simulink model "jam1722"  (R2016a)
settings: Solver=ode23tb  StartTime=0.0  StopTime=2  MaxStep=1e-4  RelTol=1e-3
undefined symbols (not defined in the file): D1, Delta
libraries: powerlib x64, sps_avr x4
settings Model: Creator=eka  LastModifiedBy=willi
settings DataIOCC: SaveFormat=StructureWithTime
settings DebuggingCC: UnconnectedInputMsg=none  UnconnectedOutputMsg=none  UnconnectedLineMsg=none
settings HardwareCC: ProdWordSize=32  ProdHWDeviceType=Specified
settings ConfigComp: CovModelRefEnable=Off

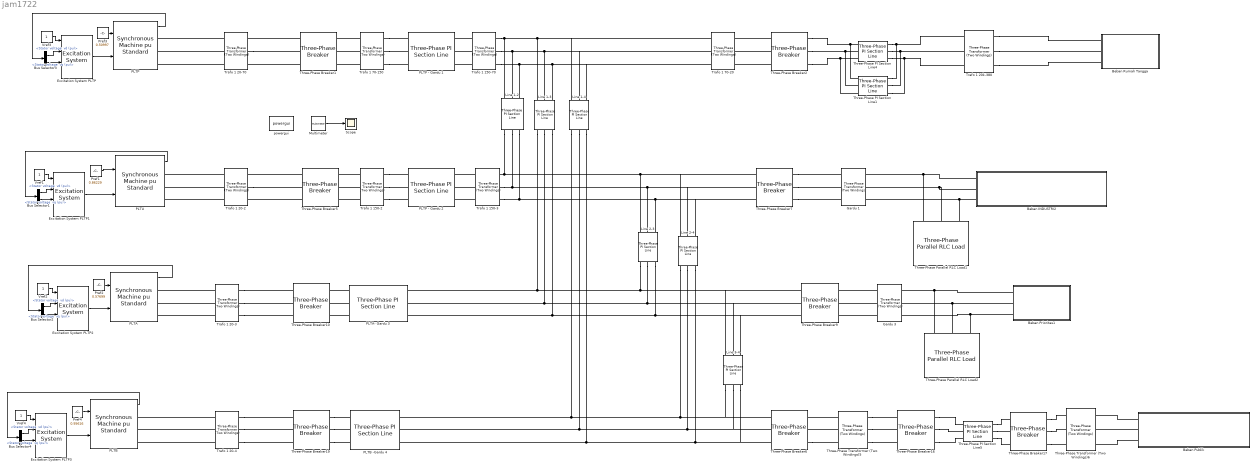
== system jam1722 ==
  Beban INDUSTRI2 : Subsystem
  Beban Prioritas1 : Subsystem
  Beban Publik : Subsystem
  Beban Rumah Tangga : Subsystem
  Bus Selector{1..4} (4 alike) : BusSelector  OutputSignals="dq0 components.Stator voltage  vd (pu),dq0 components.Stator voltage  vq (pu)"
  Excitation System PLTP : sps_avr/Excitation System  tr=20e-3  reg=[ 300, 0.001 ]  exc=[ 1, 0 ]  tgr=[ 0, 0 ]  damp=[ 0.001, 0.1 ]  sat=[ 0, 0 ]  lim=[ -11.5, 11.5, 0 ]  v0=[1 1.2849]
  Excitation System PLTP1 : sps_avr/Excitation System  tr=20e-3  reg=[ 300, 0.001 ]  exc=[ 1, 0 ]  tgr=[ 0, 0 ]  damp=[ 0.001, 0.1 ]  sat=[ 0, 0 ]  lim=[ -11.5, 11.5, 0 ]  v0=[1 1.6958]
  Excitation System PLTP2 : sps_avr/Excitation System  tr=20e-3  reg=[ 300, 0.001 ]  exc=[ 1, 0 ]  tgr=[ 0, 0 ]  damp=[ 0.001, 0.1 ]  sat=[ 0, 0 ]  lim=[ -11.5, 11.5, 0 ]  v0=[1 1.4349]
  Excitation System PLTP3 : sps_avr/Excitation System  tr=20e-3  reg=[ 300, 0.001 ]  exc=[ 1, 0 ]  tgr=[ 0, 0 ]  damp=[ 0.001, 0.1 ]  sat=[ 0, 0 ]  lim=[ -11.5, 11.5, 0 ]  v0=[1 4.931]
  Gardu 1 : powerlib/Elements/Three-Phase Transformer (Two Windings)  Winding1Connection=Yg  Winding2Connection=Delta (D1)  CoreType=Three single-phase transformers  SetSaturation=off  Hysteresis=off  DataFile='hysteresis'  SetInitialFlux=off  Measurements=None  UNITS=pu  NominalPower=[ 250e6 , 50 ]  Winding1=[ 70e3 , 0.005 , 0.0159 ]  Winding2=[ 20e3 , 0.005 , 0]  Rm=500  Lm=500  L0=0.5  Saturation=[ 0,0 ; 0.0024,1.2 ; 1.0,1.52 ]  InitialFluxes=[ 0.8 , -0.8 , 0.7 ]  MoreParameters=off  BreakLoop=off  DataType=off  TransfoNumber=1
  Gardu 3 : powerlib/Elements/Three-Phase Transformer (Two Windings)  Winding1Connection=Yg  Winding2Connection=Delta (D1)  CoreType=Three single-phase transformers  SetSaturation=off  Hysteresis=off  DataFile='hysteresis'  SetInitialFlux=off  Measurements=None  UNITS=pu  NominalPower=[ 250e6 , 50 ]  Winding1=[ 70e3 , 0.005 , 0.0159 ]  Winding2=[20e3 , 0.005 , 0]  Rm=500  Lm=500  L0=0.5  Saturation=[ 0,0 ; 0.0024,1.2 ; 1.0,1.52 ]  InitialFluxes=[ 0.8 , -0.8 , 0.7 ]  MoreParameters=off  BreakLoop=off  DataType=off  TransfoNumber=1
  Line 1-2 : powerlib/Elements/Three-Phase PI Section Line  LConnTagsString=a|b|c  RConnTagsString=A|B|C  Frequency=50  Resistances=[ 0.2 0.3864]  Inductances="[ 0.9337e-3  4.1264e-3]"  Capacitances=[12.74e-9 7.751e-9]  Length=20
  Line 1-3 : powerlib/Elements/Three-Phase PI Section Line  LConnTagsString=a|b|c  RConnTagsString=A|B|C  Frequency=50  Resistances=[ 0.2 0.3864]  Inductances="[ 0.9337e-3  4.1264e-3]"  Capacitances=[12.74e-9 7.751e-9]  Length=5
  Line 1-4 : powerlib/Elements/Three-Phase PI Section Line  LConnTagsString=a|b|c  RConnTagsString=A|B|C  Frequency=50  Resistances=[ 0.2 0.3864]  Inductances="[ 0.9337e-3  4.1264e-3]"  Capacitances=[12.74e-9 7.751e-9]  Length=20
  Line 2-3 : powerlib/Elements/Three-Phase PI Section Line  LConnTagsString=a|b|c  RConnTagsString=A|B|C  Frequency=50  Resistances=[ 0.2 0.3864]  Inductances="[ 0.9337e-3  4.1264e-3]"  Capacitances=[12.74e-9 7.751e-9]  Length=5
  Line 2-4 : powerlib/Elements/Three-Phase PI Section Line  LConnTagsString=a|b|c  RConnTagsString=A|B|C  Frequency=50  Resistances=[ 0.2 0.3864]  Inductances="[ 0.9337e-3  4.1264e-3]"  Capacitances=[12.74e-9 7.751e-9]  Length=20
  Line 3-4 : powerlib/Elements/Three-Phase PI Section Line  LConnTagsString=a|b|c  RConnTagsString=A|B|C  Frequency=50  Resistances=[ 0.2 0.3864]  Inductances="[ 0.9337e-3  4.1264e-3]"  Capacitances=[12.74e-9 7.751e-9]  Length=5
  Multimeter : powerlib/Measurements/Multimeter  PhasorSimulation=off  OutputType=Complex  sel=1  L=1  Gain=0  yselected={}  PSBOutputType=1  PSBequivalent=0  AxesSetting=[0,0.1,-100,100]  Display=0  SavedBlockNames=-11
  PLTA : powerlib/Machines/Synchronous Machine pu Standard  PresetModel=No  MechanicalLoad=Mechanical power Pm  ShowDetailedParameters=on  RotorType=Salient-pole  Units=per unit standard parameters  MeasurementBus=off  NominalParameters=[36e6 20000 50]  Reactances1=[ 1.81, 0.3, 0.23, 1.76, 0.65, 0.25, 0.15 ]  Reactances2=[2.24 0.17 0.12 1.02 0.13 0.08]  dAxisTimeConstants=Short-circuit  qAxisTimeConstants=Short-circuit  TimeConstants1="[ 4.4849  0.0681  0.1  ]"  TimeConstants2=[ 8.0, 0.03, 1.0, 0.07 ]  TimeConstants3="[  4.49  0.0681  0.0513  ]"  TimeConstants4=[ 8.0, 0.03, 0.3371, 0.0295 ]  TimeConstants5=[ 1.01, 0.053, 0.1 ]  TimeConstants6=[ 1.3201, 0.023, 1.0, 0.07 ]  TimeConstants7=[0.012 0.003 0.003]  TimeConstants8=[ 1.3201, 0.0231, 0.3371, 0.0295 ]  StatorResistance=0.037875  Mechanical=[0.1028 0.02056 2]  PolePairs=2  InitialConditions=[0 -59.3108 0.566752 0.566752 0.566752 4.73334 -115.267 124.733 1.43489]  SetSaturation=on  Saturation=[0.6404,0.7127,0.8441,0.9214,0.9956,1.082,1.19,1.316,1.457;0.7,0.7698,0.8872,0.9466,0.9969,1.046,1.1,1.151,1.201]  LoadFlowParameters=[1,0,0,0,0]  TsPowergui=0  TsBlock=-1  IterativeModel=Trapezoidal non iterative  IterativeDiscreteModel=Trapezoidal non iterative  BusType=swing  Pref=0  Qref=0  Qmin=-inf  Qmax=inf  PLF=0  QLF=0
  PLTA- Gardu 3 : powerlib/Elements/Three-Phase PI Section Line  LConnTagsString=a|b|c  RConnTagsString=A|B|C  Frequency=50  Resistances=[ 0.2 0.3864]  Inductances="[ 0.9337e-3  4.1264e-3]"  Capacitances=[12.74e-9 7.751e-9]  Length=50
  PLTB : powerlib/Machines/Synchronous Machine pu Standard  PresetModel=No  MechanicalLoad=Mechanical power Pm  ShowDetailedParameters=on  RotorType=Salient-pole  Units=per unit standard parameters  MeasurementBus=off  NominalParameters=[12e6 20000 50]  Reactances1=[ 1.81, 0.3, 0.23, 1.76, 0.65, 0.25, 0.15 ]  Reactances2=[2.24 0.17 0.12 1.02 0.13 0.08]  dAxisTimeConstants=Short-circuit  qAxisTimeConstants=Short-circuit  TimeConstants1="[ 4.4849  0.0681  0.1  ]"  TimeConstants2=[ 8.0, 0.03, 1.0, 0.07 ]  TimeConstants3="[  4.49  0.0681  0.0513  ]"  TimeConstants4=[ 8.0, 0.03, 0.3371, 0.0295 ]  TimeConstants5=[ 1.01, 0.053, 0.1 ]  TimeConstants6=[ 1.3201, 0.023, 1.0, 0.07 ]  TimeConstants7=[0.012 0.003 0.003]  TimeConstants8=[ 1.3201, 0.0231, 0.3371, 0.0295 ]  StatorResistance=0.037875  Mechanical=[0.1028 0.02056 2]  PolePairs=2  InitialConditions=[0 -77.6086 1.80081 1.80081 1.80081 -66.5761 -186.576 53.4239 4.93097]  SetSaturation=on  Saturation=[0.6404,0.7127,0.8441,0.9214,0.9956,1.082,1.19,1.316,1.457;0.7,0.7698,0.8872,0.9466,0.9969,1.046,1.1,1.151,1.201]  LoadFlowParameters=[1,0,0,0,0]  TsPowergui=0  TsBlock=-1  IterativeModel=Trapezoidal non iterative  IterativeDiscreteModel=Trapezoidal non iterative  BusType=PV  Pref=10e6  Qref=0  Qmin=-inf  Qmax=inf  PLF=0  QLF=0
  PLTB -Gardu 4 : powerlib/Elements/Three-Phase PI Section Line  LConnTagsString=a|b|c  RConnTagsString=A|B|C  Frequency=50  Resistances=[ 0.2 0.3864]  Inductances="[ 0.9337e-3  4.1264e-3]"  Capacitances=[12.74e-9 7.751e-9]  Length=20
  PLTP : powerlib/Machines/Synchronous Machine pu Standard  PresetModel=No  MechanicalLoad=Mechanical power Pm  ShowDetailedParameters=on  RotorType=Salient-pole  Units=per unit standard parameters  MeasurementBus=off  NominalParameters=[96e6 20000 50]  Reactances1=[ 1.81, 0.3, 0.23, 1.76, 0.65, 0.25, 0.15 ]  Reactances2=[2.24 0.17 0.12 1.02 0.13 0.08]  dAxisTimeConstants=Short-circuit  qAxisTimeConstants=Short-circuit  TimeConstants1="[ 4.4849  0.0681  0.1  ]"  TimeConstants2=[ 8.0, 0.03, 1.0, 0.07 ]  TimeConstants3="[  4.49  0.0681  0.0513  ]"  TimeConstants4=[ 8.0, 0.03, 0.3371, 0.0295 ]  TimeConstants5=[ 1.01, 0.053, 0.1 ]  TimeConstants6=[ 1.3201, 0.023, 1.0, 0.07 ]  TimeConstants7=[0.012 0.003 0.003]  TimeConstants8=[ 1.3201, 0.0231, 0.3371, 0.0295 ]  StatorResistance=0.037875  Mechanical=[0.1028 0.02056 2]  PolePairs=2  InitialConditions=[0 -61.4393 0.505842 0.505842 0.505842 8.5019 -111.498 128.502 1.28494]  SetSaturation=on  Saturation=[0.6404,0.7127,0.8441,0.9214,0.9956,1.082,1.19,1.316,1.457;0.7,0.7698,0.8872,0.9466,0.9969,1.046,1.1,1.151,1.201]  LoadFlowParameters=[1,0,0,0,0]  TsPowergui=0  TsBlock=-1  IterativeModel=Trapezoidal non iterative  IterativeDiscreteModel=Trapezoidal non iterative  BusType=swing  Pref=400E6  Qref=0  Qmin=-inf  Qmax=inf  PLF=0  QLF=0
  PLTP - Gardu 1 : powerlib/Elements/Three-Phase PI Section Line  LConnTagsString=a|b|c  RConnTagsString=A|B|C  Frequency=50  Resistances=[ 0.2 0.3864]  Inductances="[ 0.9337e-3  4.1264e-3]"  Capacitances=[12.74e-9 7.751e-9]  Length=100
  PLTP - Gardu 2 : powerlib/Elements/Three-Phase PI Section Line  LConnTagsString=a|b|c  RConnTagsString=A|B|C  Frequency=50  Resistances=[ 0.2 0.3864]  Inductances="[ 0.9337e-3  4.1264e-3]"  Capacitances=[12.74e-9 7.751e-9]  Length=100
  PLTU : powerlib/Machines/Synchronous Machine pu Standard  PresetModel=No  MechanicalLoad=Mechanical power Pm  ShowDetailedParameters=on  RotorType=Salient-pole  Units=per unit standard parameters  MeasurementBus=off  NominalParameters=[120e6 20000 50]  Reactances1=[ 1.81, 0.3, 0.23, 1.76, 0.65, 0.25, 0.15 ]  Reactances2=[2.24 0.17 0.12 1.02 0.13 0.08]  dAxisTimeConstants=Short-circuit  qAxisTimeConstants=Short-circuit  TimeConstants1="[ 4.4849  0.0681  0.1  ]"  TimeConstants2=[ 8.0, 0.03, 1.0, 0.07 ]  TimeConstants3="[  4.49  0.0681  0.0513  ]"  TimeConstants4=[ 8.0, 0.03, 0.3371, 0.0295 ]  TimeConstants5=[ 1.01, 0.053, 0.1 ]  TimeConstants6=[ 1.3201, 0.023, 1.0, 0.07 ]  TimeConstants7=[0.012 0.003 0.003]  TimeConstants8=[ 1.3201, 0.0231, 0.3371, 0.0295 ]  StatorResistance=0.037875  Mechanical=[0.1028 0.02056 2]  PolePairs=2  InitialConditions=[0 -93.9732 0.874366 0.874366 0.874366 -34.8255 -154.826 85.1745 1.69579]  SetSaturation=on  Saturation=[0.6404,0.7127,0.8441,0.9214,0.9956,1.082,1.19,1.316,1.457;0.7,0.7698,0.8872,0.9466,0.9969,1.046,1.1,1.151,1.201]  LoadFlowParameters=[1,0,0,0,0]  TsPowergui=0  TsBlock=-1  IterativeModel=Trapezoidal non iterative  IterativeDiscreteModel=Trapezoidal non iterative  BusType=PV  Pref=100e6  Qref=0  Qmin=-inf  Qmax=inf  PLF=0  QLF=0
  Pref1 : Constant  Value=0.86229
  Pref2 : Constant  Value=0.57699
  Pref3 : Constant  Value=0.50997
  Pref4 : Constant  Value=0.95616
  Scope : Scope
  Three-Phase PI Section Line1 : powerlib/Elements/Three-Phase PI Section Line  LConnTagsString=a|b|c  RConnTagsString=A|B|C  Frequency=50  Resistances=[ 0.2 0.3864]  Inductances="[ 0.9337e-3  4.1264e-3]"  Capacitances=[12.74e-9 7.751e-9]  Length=3
  Three-Phase PI Section Line4 : powerlib/Elements/Three-Phase PI Section Line  LConnTagsString=a|b|c  RConnTagsString=A|B|C  Frequency=50  Resistances=[ 0.2 0.3864]  Inductances="[ 0.9337e-3  4.1264e-3]"  Capacitances=[12.74e-9 7.751e-9]  Length=3
  Three-Phase PI Section Line5 : powerlib/Elements/Three-Phase PI Section Line  LConnTagsString=a|b|c  RConnTagsString=A|B|C  Frequency=50  Resistances=[ 0.2 0.3864]  Inductances="[ 0.9337e-3  4.1264e-3]"  Capacitances=[12.74e-9 7.751e-9]  Length=3
  Three-Phase Parallel RLC Load1 : powerlib/Elements/Three-Phase Parallel RLC Load  LConnTagsString=A|B|C  Configuration=Delta  NominalVoltage=380  Vabc=[1e3 1e3 1e3]  Vabcp=[1e3 1e3 1e3]  NominalFrequency=50  UnbalancedPower=off  ActivePower=0  InductivePower=0  CapacitivePower=35000  Pabc=[10e3 9e3 11e3]  QLabc=[100 90 110]  QCabc=[100 90 110]  Pabcp=[10e3 9e3 11e3]  QLabcp=[100 90 110]  QCabcp=[100 90 110]  Measurements=None  LoadType=constant Z
  Three-Phase Parallel RLC Load2 : powerlib/Elements/Three-Phase Parallel RLC Load  LConnTagsString=A|B|C  Configuration=Delta  NominalVoltage=380  Vabc=[1e3 1e3 1e3]  Vabcp=[1e3 1e3 1e3]  NominalFrequency=50  UnbalancedPower=off  ActivePower=0  InductivePower=0  CapacitivePower=10000  Pabc=[10e3 9e3 11e3]  QLabc=[100 90 110]  QCabc=[100 90 110]  Pabcp=[10e3 9e3 11e3]  QLabcp=[100 90 110]  QCabcp=[100 90 110]  Measurements=None  LoadType=constant Z
  Three-Phase Transformer (Two Windings)5 : powerlib/Elements/Three-Phase Transformer (Two Windings)  Winding1Connection=Delta (D1)  Winding2Connection=Yg  CoreType=Three single-phase transformers  SetSaturation=off  Hysteresis=off  DataFile='hysteresis'  SetInitialFlux=off  Measurements=None  UNITS=pu  NominalPower=[ 250e6 , 50 ]  Winding1=[70e3 , 0.005 , 0 ]  Winding2=[20e3 , 0.005 , 0.0159 ]  Rm=500  Lm=500  L0=0.5  Saturation=[ 0,0 ; 0.0024,1.2 ; 1.0,1.52 ]  InitialFluxes=[ 0.8 , -0.8 , 0.7 ]  MoreParameters=off  BreakLoop=off  DataType=off  TransfoNumber=1
  Three-Phase Transformer (Two Windings)6 : powerlib/Elements/Three-Phase Transformer (Two Windings)  Winding1Connection=Yg  Winding2Connection=Delta (D1)  CoreType=Three single-phase transformers  SetSaturation=off  Hysteresis=off  DataFile='hysteresis'  SetInitialFlux=off  Measurements=None  UNITS=pu  NominalPower=[ 220e6 , 50 ]  Winding1=[ 20e3 , 0.005 , 0.0159 ]  Winding2=[ 380 , 0.005 , 0]  Rm=500  Lm=500  L0=0.5  Saturation=[ 0,0 ; 0.0024,1.2 ; 1.0,1.52 ]  InitialFluxes=[ 0.8 , -0.8 , 0.7 ]  MoreParameters=off  BreakLoop=off  DataType=off  TransfoNumber=1
  Three-Phase Breaker{1,5..7,9..10,16..17,19} (9 alike) : powerlib/Elements/Three-Phase Breaker  InitialState=closed  SwitchA=off  SwitchB=off  SwitchC=off  SwitchTimes="[1/60  5/60]"  External=off  BreakerResistance=0.01  SnubberResistance=1e6  SnubberCapacitance=inf  Measurements=None
  Three-Phase Breaker2 : powerlib/Elements/Three-Phase Breaker  InitialState=closed  SwitchA=off  SwitchB=off  SwitchC=off  SwitchTimes="[1/60  5/60]"  External=off  BreakerResistance=0.0005  SnubberResistance=1e6  SnubberCapacitance=inf  Measurements=None
  Trafo 1 150-2 : powerlib/Elements/Three-Phase Transformer (Two Windings)  Winding1Connection=Yg  Winding2Connection=Delta (D1)  CoreType=Three single-phase transformers  SetSaturation=off  Hysteresis=off  DataFile='hysteresis'  SetInitialFlux=off  Measurements=None  UNITS=pu  NominalPower=[ 250e6 , 50 ]  Winding1=[70e3 , 0.005 , 0]  Winding2="[150e3 , 0.005 , 0.0159  ]"  Rm=500  Lm=500  L0=0.5  Saturation=[ 0,0 ; 0.0024,1.2 ; 1.0,1.52 ]  InitialFluxes=[ 0.8 , -0.8 , 0.7 ]  MoreParameters=off  BreakLoop=off  DataType=off  TransfoNumber=1
  Trafo 1 150-3 : powerlib/Elements/Three-Phase Transformer (Two Windings)  Winding1Connection=Delta (D1)  Winding2Connection=Yg  CoreType=Three single-phase transformers  SetSaturation=off  Hysteresis=off  DataFile='hysteresis'  SetInitialFlux=off  Measurements=None  UNITS=pu  NominalPower=[ 250e6 , 50 ]  Winding1=[150e3 , 0.005 , 0.0159 ]  Winding2=[70e3 , 0.005 , 0 ]  Rm=500  Lm=500  L0=0.5  Saturation=[ 0,0 ; 0.0024,1.2 ; 1.0,1.52 ]  InitialFluxes=[ 0.8 , -0.8 , 0.7 ]  MoreParameters=off  BreakLoop=off  DataType=off  TransfoNumber=1
  Trafo 1 150-70 : powerlib/Elements/Three-Phase Transformer (Two Windings)  Winding1Connection=Yg  Winding2Connection=Delta (D1)  CoreType=Three single-phase transformers  SetSaturation=off  Hysteresis=off  DataFile='hysteresis'  SetInitialFlux=off  Measurements=None  UNITS=pu  NominalPower=[ 250e6 , 50 ]  Winding1=[150e3 , 0.005 , 0.0159 ]  Winding2=[70e3 , 0.005 , 0 ]  Rm=500  Lm=500  L0=0.5  Saturation=[ 0,0 ; 0.0024,1.2 ; 1.0,1.52 ]  InitialFluxes=[ 0.8 , -0.8 , 0.7 ]  MoreParameters=off  BreakLoop=off  DataType=off  TransfoNumber=1
  Trafo 1 20-2 : powerlib/Elements/Three-Phase Transformer (Two Windings)  Winding1Connection=Delta (D1)  Winding2Connection=Yg  CoreType=Three single-phase transformers  SetSaturation=off  Hysteresis=off  DataFile='hysteresis'  SetInitialFlux=off  Measurements=None  UNITS=pu  NominalPower=[ 210e6 , 50 ]  Winding1=[20e3 , 0.005 , 0.0159 ]  Winding2=[70e3 , 0.005 , 0 ]  Rm=500  Lm=500  L0=0.5  Saturation=[ 0,0 ; 0.0024,1.2 ; 1.0,1.52 ]  InitialFluxes=[ 0.8 , -0.8 , 0.7 ]  MoreParameters=off  BreakLoop=off  DataType=off  TransfoNumber=1
  Trafo 1 20-3 : powerlib/Elements/Three-Phase Transformer (Two Windings)  Winding1Connection=Yg  Winding2Connection=Delta (D1)  CoreType=Three single-phase transformers  SetSaturation=off  Hysteresis=off  DataFile='hysteresis'  SetInitialFlux=off  Measurements=None  UNITS=pu  NominalPower=[ 210e6 , 50 ]  Winding1=[20e3 , 0.005 , 0.0159 ]  Winding2=[70e3 , 0.005 , 0 ]  Rm=500  Lm=500  L0=0.5  Saturation=[ 0,0 ; 0.0024,1.2 ; 1.0,1.52 ]  InitialFluxes=[ 0.8 , -0.8 , 0.7 ]  MoreParameters=off  BreakLoop=off  DataType=off  TransfoNumber=1
  Trafo 1 20-4 : powerlib/Elements/Three-Phase Transformer (Two Windings)  Winding1Connection=Yg  Winding2Connection=Delta (D1)  CoreType=Three single-phase transformers  SetSaturation=off  Hysteresis=off  DataFile='hysteresis'  SetInitialFlux=off  Measurements=None  UNITS=pu  NominalPower=[ 210e6 , 50 ]  Winding1=[20e3 , 0.005 , 0.0159 ]  Winding2=[70e3 , 0.005 , 0 ]  Rm=500  Lm=500  L0=0.5  Saturation=[ 0,0 ; 0.0024,1.2 ; 1.0,1.52 ]  InitialFluxes=[ 0.8 , -0.8 , 0.7 ]  MoreParameters=off  BreakLoop=off  DataType=off  TransfoNumber=1
  Trafo 1 20-70 : powerlib/Elements/Three-Phase Transformer (Two Windings)  Winding1Connection=Yg  Winding2Connection=Delta (D1)  CoreType=Three single-phase transformers  SetSaturation=off  Hysteresis=off  DataFile='hysteresis'  SetInitialFlux=off  Measurements=None  UNITS=pu  NominalPower=[ 210e6 , 50 ]  Winding1=[20e3 , 0.005 , 0.0159 ]  Winding2=[70e3 , 0.005 , 0 ]  Rm=500  Lm=500  L0=0.5  Saturation=[ 0,0 ; 0.0024,1.2 ; 1.0,1.52 ]  InitialFluxes=[ 0.8 , -0.8 , 0.7 ]  MoreParameters=off  BreakLoop=off  DataType=off  TransfoNumber=1
  Trafo 1 20k-380 : powerlib/Elements/Three-Phase Transformer (Two Windings)  Winding1Connection=Yg  Winding2Connection=Delta (D1)  CoreType=Three single-phase transformers  SetSaturation=off  Hysteresis=off  DataFile='hysteresis'  SetInitialFlux=off  Measurements=None  UNITS=pu  NominalPower=[ 220e6 , 50 ]  Winding1="[ 18000, 0.005 ,0.0159  ]"  Winding2=[ 380 , 0.005 , 0]  Rm=500  Lm=500  L0=0.5  Saturation=[ 0,0 ; 0.0024,1.2 ; 1.0,1.52 ]  InitialFluxes=[ 0.8 , -0.8 , 0.7 ]  MoreParameters=off  BreakLoop=off  DataType=off  TransfoNumber=1
  Trafo 1 70-150 : powerlib/Elements/Three-Phase Transformer (Two Windings)  Winding1Connection=Delta (D1)  Winding2Connection=Yg  CoreType=Three single-phase transformers  SetSaturation=off  Hysteresis=off  DataFile='hysteresis'  SetInitialFlux=off  Measurements=None  UNITS=pu  NominalPower=[ 250e6 , 50 ]  Winding1=[70e3 , 0.005 , 0]  Winding2="[150e3 , 0.005 , 0.0159  ]"  Rm=500  Lm=500  L0=0.5  Saturation=[ 0,0 ; 0.0024,1.2 ; 1.0,1.52 ]  InitialFluxes=[ 0.8 , -0.8 , 0.7 ]  MoreParameters=off  BreakLoop=off  DataType=off  TransfoNumber=1
  Trafo 1 70-20 : powerlib/Elements/Three-Phase Transformer (Two Windings)  Winding1Connection=Delta (D1)  Winding2Connection=Yg  CoreType=Three single-phase transformers  SetSaturation=off  Hysteresis=off  DataFile='hysteresis'  SetInitialFlux=off  Measurements=None  UNITS=pu  NominalPower=[ 220e6 , 50 ]  Winding1=[70e3 , 0.005 , 0 ]  Winding2=[20e3 , 0.005 , 0.0159 ]  Rm=500  Lm=500  L0=0.5  Saturation=[ 0,0 ; 0.0024,1.2 ; 1.0,1.52 ]  InitialFluxes=[ 0.8 , -0.8 , 0.7 ]  MoreParameters=off  BreakLoop=off  DataType=off  TransfoNumber=1
  Vref{1..4} (4 alike) : Constant
  powergui : powerlib/powergui  Priority=1  SimulationMode=Continuous  SolverType=Tustin  SampleTime=50e-6  frequency=60  SPID=on  DisableSnubberDevices=off  DisableRonSwitches=off  DisableVfSwitches=off  SwTol=0  DisplayEquations=off  Interpol=off  ExternalGateDelay=off  methode=off  Ts=100  FunctionMessages=off  echomessages=off  HookPort=off  EnableUseOfTLC=off  x0status=blocks  frequencyindice=50  Pbase=100e6  ErrMax=0.0001  Iterations=300  UnitsV=kV  UnitsW=MW  buscounter=0  RestoreLinks=warning  ResistiveCurrentMeasurement=off  Frange=[0:2:500]  Ylog=off  Xlog=on  ShowGrid=off  save=off  variable=ZData  structure=0  ZoomFFT=off  StartTime=0.0  cycles=1  DisplayStyle=1  fundamental=60  FreqAxis=off  MaxFrequency=1000  frequencyindicesteady=1  RmsSteady=1  display=off
  wires:
  Vref3/1 -> Excitation System PLTP/1
  Bus Selector3/1 -> Excitation System PLTP/2  "<Stator voltage  vd (pu)>"
  Bus Selector3/2 -> Excitation System PLTP/3  "<Stator voltage  vq (pu)>"
  Excitation System PLTP/1 -> PLTP/2
  PLTP/1 -> Bus Selector3/1
  Pref3/1 -> PLTP/1
  Vref1/1 -> Excitation System PLTP1/1
  Bus Selector1/1 -> Excitation System PLTP1/2  "<Stator voltage  vd (pu)>"
  Bus Selector1/2 -> Excitation System PLTP1/3  "<Stator voltage  vq (pu)>"
  Excitation System PLTP1/1 -> PLTU/2
  PLTU/1 -> Bus Selector1/1
  Pref1/1 -> PLTU/1
  Vref2/1 -> Excitation System PLTP2/1
  Bus Selector2/1 -> Excitation System PLTP2/2  "<Stator voltage  vd (pu)>"
  Bus Selector2/2 -> Excitation System PLTP2/3  "<Stator voltage  vq (pu)>"
  Excitation System PLTP2/1 -> PLTA/2
  PLTA/1 -> Bus Selector2/1
  Pref2/1 -> PLTA/1
  Vref4/1 -> Excitation System PLTP3/1
  Bus Selector4/1 -> Excitation System PLTP3/2  "<Stator voltage  vd (pu)>"
  Bus Selector4/2 -> Excitation System PLTP3/3  "<Stator voltage  vq (pu)>"
  Excitation System PLTP3/1 -> PLTB/2
  PLTB/1 -> Bus Selector4/1
  Pref4/1 -> PLTB/1
  Multimeter/1 -> Scope/1
  connections:
  Line 1-2/RConn1 -- Three-Phase Breaker7/LConn1 -- Line 2-4/LConn1 -- Line 2-3/LConn1 -- Trafo 1 150-3/RConn1
  Line 1-3/RConn1 -- Line 3-4/LConn1 -- Three-Phase Breaker9/LConn1 -- Line 2-3/RConn1 -- PLTA- Gardu 3/RConn1
  Line 1-3/RConn2 -- Three-Phase Breaker9/LConn2 -- Line 3-4/LConn2 -- Line 2-3/RConn2 -- PLTA- Gardu 3/RConn2
  Line 1-3/RConn3 -- Line 3-4/LConn3 -- Three-Phase Breaker9/LConn3 -- Line 2-3/RConn3 -- PLTA- Gardu 3/RConn3
  Line 1-4/RConn1 -- Line 3-4/RConn1 -- Three-Phase Breaker6/LConn1 -- Line 2-4/RConn1 -- PLTB -Gardu 4/RConn1
  Line 1-4/RConn2 -- Three-Phase Breaker6/LConn2 -- Line 3-4/RConn2 -- Line 2-4/RConn2 -- PLTB -Gardu 4/RConn2
  Line 1-4/RConn3 -- Line 3-4/RConn3 -- Three-Phase Breaker6/LConn3 -- Line 2-4/RConn3 -- PLTB -Gardu 4/RConn3
  Trafo 1 20-70/LConn1 -- PLTP/RConn1
  Trafo 1 20-70/LConn2 -- PLTP/RConn2
  Trafo 1 20-70/LConn3 -- PLTP/RConn3
  Three-Phase Breaker1/LConn1 -- Trafo 1 20-70/RConn1
  Three-Phase Breaker1/LConn3 -- Trafo 1 20-70/RConn3
  Line 1-2/LConn2 -- Trafo 1 70-20/LConn2 -- Line 1-4/LConn2 -- Line 1-3/LConn2 -- Trafo 1 150-70/RConn2
  Line 1-2/LConn1 -- Trafo 1 150-70/RConn1 -- Trafo 1 70-20/LConn1 -- Line 1-4/LConn1 -- Line 1-3/LConn1
  Line 1-2/LConn3 -- Trafo 1 70-20/LConn3 -- Line 1-4/LConn3 -- Line 1-3/LConn3 -- Trafo 1 150-70/RConn3
  Three-Phase PI Section Line4/RConn1 -- Three-Phase PI Section Line1/RConn1 -- Trafo 1 20k-380/LConn1
  Three-Phase PI Section Line4/RConn2 -- Three-Phase PI Section Line1/RConn2 -- Trafo 1 20k-380/LConn2
  Three-Phase PI Section Line4/RConn3 -- Three-Phase PI Section Line1/RConn3 -- Trafo 1 20k-380/LConn3
  Line 1-2/RConn3 -- Line 2-4/LConn3 -- Three-Phase Breaker7/LConn3 -- Line 2-3/LConn3 -- Trafo 1 150-3/RConn3
  Line 1-2/RConn2 -- Three-Phase Breaker7/LConn2 -- Line 2-4/LConn2 -- Line 2-3/LConn2 -- Trafo 1 150-3/RConn2
  Beban INDUSTRI2/LConn1 -- Gardu 1/RConn1 -- Three-Phase Parallel RLC Load1/LConn1
  Beban INDUSTRI2/LConn2 -- Gardu 1/RConn2 -- Three-Phase Parallel RLC Load1/LConn2
  Beban INDUSTRI2/LConn3 -- Gardu 1/RConn3 -- Three-Phase Parallel RLC Load1/LConn3
  Trafo 1 20-3/RConn2 -- Three-Phase Breaker10/LConn2
  Trafo 1 20-3/RConn1 -- Three-Phase Breaker10/LConn1
  Trafo 1 20-3/RConn3 -- Three-Phase Breaker10/LConn3
  PLTA- Gardu 3/LConn1 -- Three-Phase Breaker10/RConn1
  PLTA- Gardu 3/LConn2 -- Three-Phase Breaker10/RConn2
  PLTA- Gardu 3/LConn3 -- Three-Phase Breaker10/RConn3
  Three-Phase Transformer (Two Windings)5/LConn1 -- Three-Phase Breaker6/RConn1
  Three-Phase Transformer (Two Windings)5/LConn2 -- Three-Phase Breaker6/RConn2
  Three-Phase Breaker6/RConn3 -- Three-Phase Transformer (Two Windings)5/LConn3
  Three-Phase Transformer (Two Windings)5/RConn1 -- Three-Phase Breaker16/LConn1
  Three-Phase Transformer (Two Windings)5/RConn2 -- Three-Phase Breaker16/LConn2
  Three-Phase Transformer (Two Windings)5/RConn3 -- Three-Phase Breaker16/LConn3
  Three-Phase Breaker16/RConn1 -- Three-Phase PI Section Line5/LConn1
  Three-Phase Breaker16/RConn2 -- Three-Phase PI Section Line5/LConn2
  Three-Phase Breaker16/RConn3 -- Three-Phase PI Section Line5/LConn3
  Three-Phase Breaker17/RConn1 -- Three-Phase Transformer (Two Windings)6/LConn1
  Three-Phase PI Section Line5/RConn1 -- Three-Phase Breaker17/LConn1
  Three-Phase PI Section Line5/RConn2 -- Three-Phase Breaker17/LConn2
  Three-Phase PI Section Line5/RConn3 -- Three-Phase Breaker17/LConn3
  Three-Phase Breaker17/RConn2 -- Three-Phase Transformer (Two Windings)6/LConn2
  Three-Phase Breaker17/RConn3 -- Three-Phase Transformer (Two Windings)6/LConn3
  Beban Publik/LConn1 -- Three-Phase Transformer (Two Windings)6/RConn1
  Beban Publik/LConn2 -- Three-Phase Transformer (Two Windings)6/RConn2
  Beban Publik/LConn3 -- Three-Phase Transformer (Two Windings)6/RConn3
  Trafo 1 20k-380/RConn1 -- Beban Rumah Tangga/LConn1
  Trafo 1 20k-380/RConn2 -- Beban Rumah Tangga/LConn2
  Trafo 1 20k-380/RConn3 -- Beban Rumah Tangga/LConn3
  Trafo 1 20-4/RConn1 -- Three-Phase Breaker19/LConn1
  Trafo 1 20-4/RConn2 -- Three-Phase Breaker19/LConn2
  Trafo 1 20-4/RConn3 -- Three-Phase Breaker19/LConn3
  Three-Phase Breaker19/RConn3 -- PLTB -Gardu 4/LConn3
  Three-Phase Breaker19/RConn2 -- PLTB -Gardu 4/LConn2
  Three-Phase Breaker19/RConn1 -- PLTB -Gardu 4/LConn1
  Trafo 1 150-70/LConn1 -- PLTP - Gardu 1/RConn1
  Trafo 1 150-70/LConn2 -- PLTP - Gardu 1/RConn2
  Trafo 1 150-70/LConn3 -- PLTP - Gardu 1/RConn3
  Trafo 1 70-150/LConn1 -- Three-Phase Breaker1/RConn1
  Trafo 1 70-150/LConn2 -- Three-Phase Breaker1/RConn2
  Trafo 1 70-150/LConn3 -- Three-Phase Breaker1/RConn3
  Trafo 1 70-150/RConn3 -- PLTP - Gardu 1/LConn3
  Trafo 1 70-150/RConn2 -- PLTP - Gardu 1/LConn2
  Trafo 1 70-150/RConn1 -- PLTP - Gardu 1/LConn1
  Trafo 1 150-3/LConn2 -- PLTP - Gardu 2/RConn2
  Trafo 1 150-3/LConn3 -- PLTP - Gardu 2/RConn3
  Trafo 1 150-2/RConn1 -- PLTP - Gardu 2/LConn1
  Trafo 1 20-2/LConn3 -- PLTU/RConn3
  Trafo 1 150-2/RConn2 -- PLTP - Gardu 2/LConn2
  Trafo 1 150-3/LConn1 -- PLTP - Gardu 2/RConn1
  Trafo 1 150-2/LConn1 -- Three-Phase Breaker5/RConn1
  Trafo 1 20-2/LConn1 -- PLTU/RConn1
  Trafo 1 150-2/LConn2 -- Three-Phase Breaker5/RConn2
  Trafo 1 20-2/LConn2 -- PLTU/RConn2
  Trafo 1 150-2/RConn3 -- PLTP - Gardu 2/LConn3
  Three-Phase Breaker5/LConn3 -- Trafo 1 20-2/RConn3
  Three-Phase Breaker5/LConn1 -- Trafo 1 20-2/RConn1
  Trafo 1 150-2/LConn3 -- Three-Phase Breaker5/RConn3
  Trafo 1 20-70/RConn2 -- Three-Phase Breaker1/LConn2
  Trafo 1 20-2/RConn2 -- Three-Phase Breaker5/LConn2
  Gardu 3/LConn1 -- Three-Phase Breaker9/RConn1
  Gardu 3/LConn2 -- Three-Phase Breaker9/RConn2
  Beban Prioritas1/LConn3 -- Three-Phase Parallel RLC Load2/LConn3 -- Gardu 3/RConn3
  Beban Prioritas1/LConn2 -- Three-Phase Parallel RLC Load2/LConn2 -- Gardu 3/RConn2
  Beban Prioritas1/LConn1 -- Three-Phase Parallel RLC Load2/LConn1 -- Gardu 3/RConn1
  Gardu 3/LConn3 -- Three-Phase Breaker9/RConn3
  Trafo 1 20-3/LConn1 -- PLTA/RConn1
  Trafo 1 20-3/LConn2 -- PLTA/RConn2
  Trafo 1 20-3/LConn3 -- PLTA/RConn3
  Trafo 1 20-4/LConn1 -- PLTB/RConn1
  Trafo 1 20-4/LConn2 -- PLTB/RConn2
  Trafo 1 20-4/LConn3 -- PLTB/RConn3
  Three-Phase Breaker7/RConn1 -- Gardu 1/LConn1
  Three-Phase Breaker7/RConn2 -- Gardu 1/LConn2
  Three-Phase Breaker7/RConn3 -- Gardu 1/LConn3
  Three-Phase Breaker2/LConn1 -- Trafo 1 70-20/RConn1
  Three-Phase Breaker2/LConn2 -- Trafo 1 70-20/RConn2
  Three-Phase Breaker2/LConn3 -- Trafo 1 70-20/RConn3
  Three-Phase Breaker2/RConn1 -- Three-Phase PI Section Line1/LConn1 -- Three-Phase PI Section Line4/LConn1
  Three-Phase Breaker2/RConn2 -- Three-Phase PI Section Line1/LConn2 -- Three-Phase PI Section Line4/LConn2
  Three-Phase Breaker2/RConn3 -- Three-Phase PI Section Line1/LConn3 -- Three-Phase PI Section Line4/LConn3

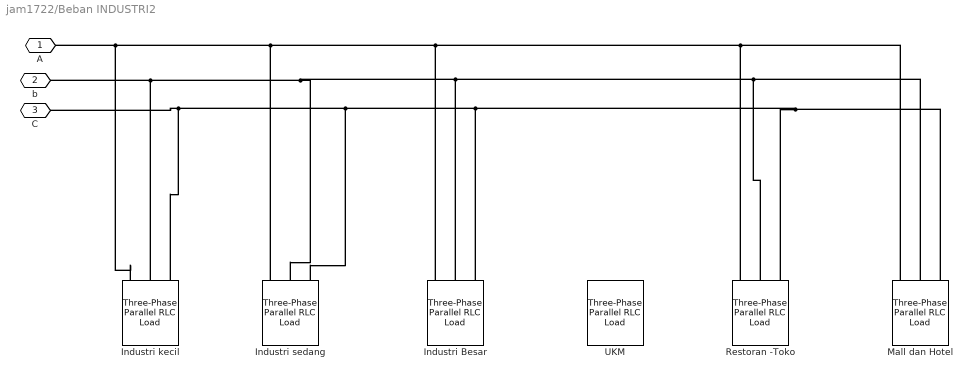
== system jam1722/Beban INDUSTRI2 ==
  Industri Besar : powerlib/Elements/Three-Phase Parallel RLC Load  LConnTagsString=A|B|C  Configuration=Delta  NominalVoltage=20000  Vabc=[1e3 1e3 1e3]  Vabcp=[1e3 1e3 1e3]  NominalFrequency=50  UnbalancedPower=off  ActivePower=8500000  InductivePower=5267826.876  CapacitivePower=0  Pabc=[10e3 9e3 11e3]  QLabc=[100 90 110]  QCabc=[100 90 110]  Pabcp=[10e3 9e3 11e3]  QLabcp=[100 90 110]  QCabcp=[100 90 110]  Measurements=None  LoadType=constant Z
  Industri kecil : powerlib/Elements/Three-Phase Parallel RLC Load  LConnTagsString=A|B|C  Configuration=Delta  NominalVoltage=20000  Vabc=[1e3 1e3 1e3]  Vabcp=[1e3 1e3 1e3]  NominalFrequency=50  UnbalancedPower=off  ActivePower=5610000  InductivePower=3476765.738  CapacitivePower=0  Pabc=[10e3 9e3 11e3]  QLabc=[100 90 110]  QCabc=[100 90 110]  Pabcp=[10e3 9e3 11e3]  QLabcp=[100 90 110]  QCabcp=[100 90 110]  Measurements=None  LoadType=constant Z
  Industri sedang : powerlib/Elements/Three-Phase Parallel RLC Load  LConnTagsString=A|B|C  Configuration=Delta  NominalVoltage=20000  Vabc=[1e3 1e3 1e3]  Vabcp=[1e3 1e3 1e3]  NominalFrequency=50  UnbalancedPower=off  ActivePower=42500000  InductivePower=26339134.38  CapacitivePower=0  Pabc=[10e3 9e3 11e3]  QLabc=[100 90 110]  QCabc=[100 90 110]  Pabcp=[10e3 9e3 11e3]  QLabcp=[100 90 110]  QCabcp=[100 90 110]  Measurements=None  LoadType=constant Z
  Mall dan Hotel : powerlib/Elements/Three-Phase Parallel RLC Load  LConnTagsString=A|B|C  Configuration=Delta  NominalVoltage=20000  Vabc=[1e3 1e3 1e3]  Vabcp=[1e3 1e3 1e3]  NominalFrequency=50  UnbalancedPower=off  ActivePower=850000  InductivePower=526782.6876  CapacitivePower=0  Pabc=[10e3 9e3 11e3]  QLabc=[100 90 110]  QCabc=[100 90 110]  Pabcp=[10e3 9e3 11e3]  QLabcp=[100 90 110]  QCabcp=[100 90 110]  Measurements=None  LoadType=constant Z
  Restoran -Toko : powerlib/Elements/Three-Phase Parallel RLC Load  LConnTagsString=A|B|C  Configuration=Delta  NominalVoltage=20000  Vabc=[1e3 1e3 1e3]  Vabcp=[1e3 1e3 1e3]  NominalFrequency=50  UnbalancedPower=off  ActivePower=4250000  InductivePower=2633913.438  CapacitivePower=0  Pabc=[10e3 9e3 11e3]  QLabc=[100 90 110]  QCabc=[100 90 110]  Pabcp=[10e3 9e3 11e3]  QLabcp=[100 90 110]  QCabcp=[100 90 110]  Measurements=None  LoadType=constant Z
  UKM : powerlib/Elements/Three-Phase Parallel RLC Load  LConnTagsString=A|B|C  Configuration=Delta  NominalVoltage=20000  Vabc=[1e3 1e3 1e3]  Vabcp=[1e3 1e3 1e3]  NominalFrequency=50  UnbalancedPower=off  ActivePower=5525000  InductivePower=3424087  CapacitivePower=0  Pabc=[10e3 9e3 11e3]  QLabc=[100 90 110]  QCabc=[100 90 110]  Pabcp=[10e3 9e3 11e3]  QLabcp=[100 90 110]  QCabcp=[100 90 110]  Measurements=None  LoadType=constant Z
  A : PMIOPort  Port=1  Side=Left
  b : PMIOPort  Port=2  Side=Left
  C : PMIOPort  Port=3  Side=Left
  connections:
  Mall dan Hotel/LConn3 -- Restoran -Toko/LConn3 -- Industri Besar/LConn3 -- Industri sedang/LConn3 -- C/RConn1 -- Industri kecil/LConn3
  A/RConn1 -- Mall dan Hotel/LConn1 -- Restoran -Toko/LConn1 -- Industri Besar/LConn1 -- Industri sedang/LConn1 -- Industri kecil/LConn1
  Mall dan Hotel/LConn2 -- Restoran -Toko/LConn2 -- Industri Besar/LConn2 -- Industri sedang/LConn2 -- Industri kecil/LConn2 -- b/RConn1

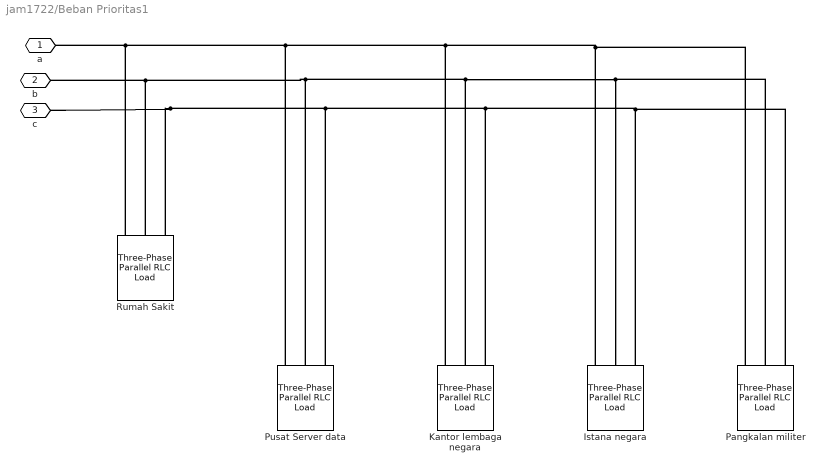
== system jam1722/Beban Prioritas1 ==
  Istana negara : powerlib/Elements/Three-Phase Parallel RLC Load  LConnTagsString=A|B|C  Configuration=Delta  NominalVoltage=20000  Vabc=[1e3 1e3 1e3]  Vabcp=[1e3 1e3 1e3]  NominalFrequency=50  UnbalancedPower=off  ActivePower=850000  InductivePower=526782.6876  CapacitivePower=0  Pabc=[10e3 9e3 11e3]  QLabc=[100 90 110]  QCabc=[100 90 110]  Pabcp=[10e3 9e3 11e3]  QLabcp=[100 90 110]  QCabcp=[100 90 110]  Measurements=None  LoadType=constant Z
  Kantor lembaga negara : powerlib/Elements/Three-Phase Parallel RLC Load  LConnTagsString=A|B|C  Configuration=Delta  NominalVoltage=20000  Vabc=[1e3 1e3 1e3]  Vabcp=[1e3 1e3 1e3]  NominalFrequency=50  UnbalancedPower=off  ActivePower=850000  InductivePower=526782.6876  CapacitivePower=0  Pabc=[10e3 9e3 11e3]  QLabc=[100 90 110]  QCabc=[100 90 110]  Pabcp=[10e3 9e3 11e3]  QLabcp=[100 90 110]  QCabcp=[100 90 110]  Measurements=None  LoadType=constant Z
  Pangkalan militer : powerlib/Elements/Three-Phase Parallel RLC Load  LConnTagsString=A|B|C  Configuration=Delta  NominalVoltage=20000  Vabc=[1e3 1e3 1e3]  Vabcp=[1e3 1e3 1e3]  NominalFrequency=50  UnbalancedPower=off  ActivePower=1912500  InductivePower=1185261.047  CapacitivePower=0  Pabc=[10e3 9e3 11e3]  QLabc=[100 90 110]  QCabc=[100 90 110]  Pabcp=[10e3 9e3 11e3]  QLabcp=[100 90 110]  QCabcp=[100 90 110]  Measurements=None  LoadType=constant Z
  Pusat Server data : powerlib/Elements/Three-Phase Parallel RLC Load  LConnTagsString=A|B|C  Configuration=Delta  NominalVoltage=20000  Vabc=[1e3 1e3 1e3]  Vabcp=[1e3 1e3 1e3]  NominalFrequency=50  UnbalancedPower=off  ActivePower=21250  InductivePower=13169.5672  CapacitivePower=0  Pabc=[10e3 9e3 11e3]  QLabc=[100 90 110]  QCabc=[100 90 110]  Pabcp=[10e3 9e3 11e3]  QLabcp=[100 90 110]  QCabcp=[100 90 110]  Measurements=None  LoadType=constant Z
  Rumah Sakit : powerlib/Elements/Three-Phase Parallel RLC Load  LConnTagsString=A|B|C  Configuration=Delta  NominalVoltage=20000  Vabc=[1e3 1e3 1e3]  Vabcp=[1e3 1e3 1e3]  NominalFrequency=50  UnbalancedPower=off  ActivePower=850000  InductivePower=526782.688  CapacitivePower=0  Pabc=[10e3 9e3 11e3]  QLabc=[100 90 110]  QCabc=[100 90 110]  Pabcp=[10e3 9e3 11e3]  QLabcp=[100 90 110]  QCabcp=[100 90 110]  Measurements=None  LoadType=constant Z
  a : PMIOPort  Port=1  Side=Left
  b : PMIOPort  Port=2  Side=Left
  c : PMIOPort  Port=3  Side=Left
  connections:
  Rumah Sakit/LConn1 -- Pangkalan militer/LConn1 -- Istana negara/LConn1 -- Kantor lembaga negara/LConn1 -- Pusat Server data/LConn1 -- a/RConn1
  b/RConn1 -- Pangkalan militer/LConn2 -- Istana negara/LConn2 -- Kantor lembaga negara/LConn2 -- Pusat Server data/LConn2 -- Rumah Sakit/LConn2
  c/RConn1 -- Pangkalan militer/LConn3 -- Istana negara/LConn3 -- Kantor lembaga negara/LConn3 -- Pusat Server data/LConn3 -- Rumah Sakit/LConn3

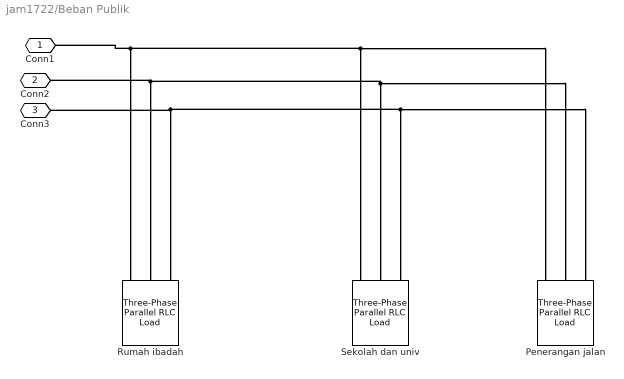
== system jam1722/Beban Publik ==
  Penerangan jalan : powerlib/Elements/Three-Phase Parallel RLC Load  LConnTagsString=A|B|C  Configuration=Delta  NominalVoltage=380  Vabc=[1e3 1e3 1e3]  Vabcp=[1e3 1e3 1e3]  NominalFrequency=50  UnbalancedPower=off  ActivePower=1700000  InductivePower=1053565.375  CapacitivePower=0  Pabc=[10e3 9e3 11e3]  QLabc=[100 90 110]  QCabc=[100 90 110]  Pabcp=[10e3 9e3 11e3]  QLabcp=[100 90 110]  QCabcp=[100 90 110]  Measurements=None  LoadType=constant Z
  Rumah ibadah : powerlib/Elements/Three-Phase Parallel RLC Load  LConnTagsString=A|B|C  Configuration=Delta  NominalVoltage=380  Vabc=[1e3 1e3 1e3]  Vabcp=[1e3 1e3 1e3]  NominalFrequency=50  UnbalancedPower=off  ActivePower=1122000  InductivePower=695353.1477  CapacitivePower=0  Pabc=[10e3 9e3 11e3]  QLabc=[100 90 110]  QCabc=[100 90 110]  Pabcp=[10e3 9e3 11e3]  QLabcp=[100 90 110]  QCabcp=[100 90 110]  Measurements=None  LoadType=constant Z
  Sekolah dan univ : powerlib/Elements/Three-Phase Parallel RLC Load  LConnTagsString=A|B|C  Configuration=Delta  NominalVoltage=380  Vabc=[1e3 1e3 1e3]  Vabcp=[1e3 1e3 1e3]  NominalFrequency=50  UnbalancedPower=off  ActivePower=850000  InductivePower=526782.6876  CapacitivePower=0  Pabc=[10e3 9e3 11e3]  QLabc=[100 90 110]  QCabc=[100 90 110]  Pabcp=[10e3 9e3 11e3]  QLabcp=[100 90 110]  QCabcp=[100 90 110]  Measurements=None  LoadType=constant Z
  Conn1 : PMIOPort  Port=1  Side=Left
  Conn2 : PMIOPort  Port=2  Side=Left
  Conn3 : PMIOPort  Port=3  Side=Left
  connections:
  Conn1/RConn1 -- Penerangan jalan/LConn1 -- Sekolah dan univ/LConn1 -- Rumah ibadah/LConn1
  Penerangan jalan/LConn2 -- Sekolah dan univ/LConn2 -- Rumah ibadah/LConn2 -- Conn2/RConn1
  Penerangan jalan/LConn3 -- Sekolah dan univ/LConn3 -- Rumah ibadah/LConn3 -- Conn3/RConn1

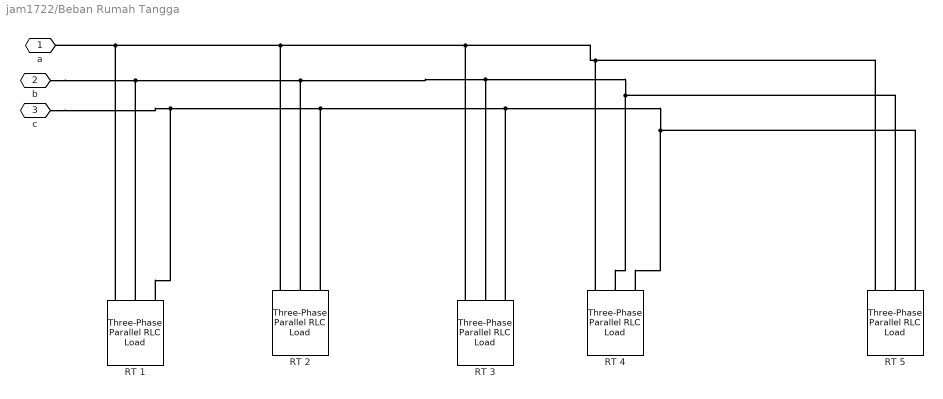
== system jam1722/Beban Rumah Tangga ==
  RT 1 : powerlib/Elements/Three-Phase Parallel RLC Load  LConnTagsString=A|B|C  Configuration=Delta  NominalVoltage=380  Vabc=[1e3 1e3 1e3]  Vabcp=[1e3 1e3 1e3]  NominalFrequency=50  UnbalancedPower=off  ActivePower=3.2175e6  InductivePower=0  CapacitivePower=0  Pabc=[10e3 9e3 11e3]  QLabc=[100 90 110]  QCabc=[100 90 110]  Pabcp=[10e3 9e3 11e3]  QLabcp=[100 90 110]  QCabcp=[100 90 110]  Measurements=None  LoadType=constant Z
  RT 2 : powerlib/Elements/Three-Phase Parallel RLC Load  LConnTagsString=A|B|C  Configuration=Delta  NominalVoltage=380  Vabc=[1e3 1e3 1e3]  Vabcp=[1e3 1e3 1e3]  NominalFrequency=50  UnbalancedPower=off  ActivePower=19.305e6  InductivePower=0  CapacitivePower=0  Pabc=[10e3 9e3 11e3]  QLabc=[100 90 110]  QCabc=[100 90 110]  Pabcp=[10e3 9e3 11e3]  QLabcp=[100 90 110]  QCabcp=[100 90 110]  Measurements=None  LoadType=constant Z
  RT 3 : powerlib/Elements/Three-Phase Parallel RLC Load  LConnTagsString=A|B|C  Configuration=Delta  NominalVoltage=380  Vabc=[1e3 1e3 1e3]  Vabcp=[1e3 1e3 1e3]  NominalFrequency=50  UnbalancedPower=off  ActivePower=47.97e6  InductivePower=0  CapacitivePower=0  Pabc=[10e3 9e3 11e3]  QLabc=[100 90 110]  QCabc=[100 90 110]  Pabcp=[10e3 9e3 11e3]  QLabcp=[100 90 110]  QCabcp=[100 90 110]  Measurements=None  LoadType=constant Z
  RT 4 : powerlib/Elements/Three-Phase Parallel RLC Load  LConnTagsString=A|B|C  Configuration=Delta  NominalVoltage=380  Vabc=[1e3 1e3 1e3]  Vabcp=[1e3 1e3 1e3]  NominalFrequency=50  UnbalancedPower=off  ActivePower=11.749e6  InductivePower=0  CapacitivePower=0  Pabc=[10e3 9e3 11e3]  QLabc=[100 90 110]  QCabc=[100 90 110]  Pabcp=[10e3 9e3 11e3]  QLabcp=[100 90 110]  QCabcp=[100 90 110]  Measurements=None  LoadType=constant Z
  RT 5 : powerlib/Elements/Three-Phase Parallel RLC Load  LConnTagsString=A|B|C  Configuration=Delta  NominalVoltage=380  Vabc=[1e3 1e3 1e3]  Vabcp=[1e3 1e3 1e3]  NominalFrequency=50  UnbalancedPower=off  ActivePower=8.7263e6  InductivePower=0  CapacitivePower=0  Pabc=[10e3 9e3 11e3]  QLabc=[100 90 110]  QCabc=[100 90 110]  Pabcp=[10e3 9e3 11e3]  QLabcp=[100 90 110]  QCabcp=[100 90 110]  Measurements=None  LoadType=constant Z
  a : PMIOPort  Port=1  Side=Left
  b : PMIOPort  Port=2  Side=Left
  c : PMIOPort  Port=3  Side=Left
  connections:
  RT 5/LConn1 -- a/RConn1 -- RT 1/LConn1 -- RT 2/LConn1 -- RT 3/LConn1 -- RT 4/LConn1
  b/RConn1 -- RT 1/LConn2 -- RT 2/LConn2 -- RT 3/LConn2 -- RT 4/LConn2 -- RT 5/LConn2
  c/RConn1 -- RT 1/LConn3 -- RT 4/LConn3 -- RT 5/LConn3 -- RT 3/LConn3 -- RT 2/LConn3
